simulink model "W1Q1"  (R2020a)
settings: Solver=VariableStepAuto  StartTime=0.0  StopTime=10  FixedStep=10  RelTol=1e-3
values from neighbouring files (symbols this model uses):
  b = 50    [para.m]
  k1 = 50    [para.m]
  k12 = 500    [para.m]
  M1 = 100    [para.m]
  m2 = 5    [para.m]
settings Model: Creator=Vinayak  LastModifiedBy=Vinayak

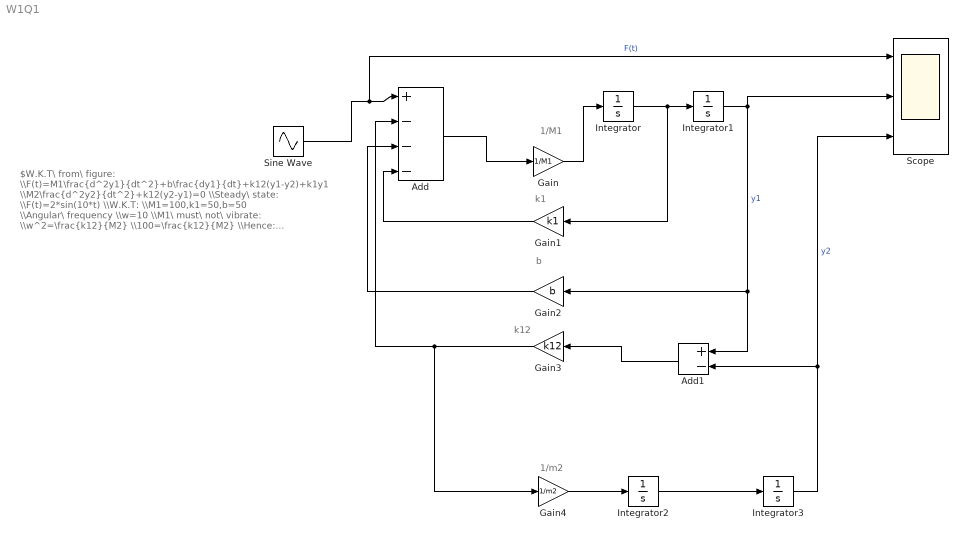
== system W1Q1 ==
  note: $W.K.T\ from\ figure: \\F(t)=M1\frac{d^2y1}{dt^2}+b\frac{dy1}{dt}+k12(y1-y2)+k1y1 \\M2\frac{d^2y2}{dt^2}+k12(y2-y1)=0 \\Steady\ state: \\F(t)=2*sin(10*t) \\W.K.T: \\M1=100,k1=50,b=50 \\Angular\ frequency \\w=10 \\M1\ must\ not\ vibrate: \\w^2=\frac{k12}{M2} \\100=\frac{k12}{M2} \\Hence: \\k12=500,M2=5.$
  note: 1/M1
  note: k1
  note: b
  note: k12
  note: 1/m2
  Add : Sum  Inputs=+---
  Add1 : Sum  Inputs=+-
  Gain : Gain  Gain=1/M1
  Gain1 : Gain  Gain=k1
  Gain2 : Gain  Gain=b
  Gain3 : Gain  Gain=k12
  Gain4 : Gain  Gain=1/m2
  Integrator{,1..3} (4 alike) : Integrator
  Scope : Scope  NumInputPorts=3
  Sine Wave : Sin  Amplitude=2  Frequency=10  SampleTime=0
  wires:
  Sine Wave/1 -> Scope/1, Add/1  "F(t)"
  Add/1 -> Gain/1
  Gain/1 -> Integrator/1
  Integrator/1 -> Gain1/1, Integrator1/1
  Gain1/1 -> Add/4
  Integrator1/1 -> Add1/1, Gain2/1, Scope/2  "y1"
  Gain2/1 -> Add/3
  Add1/1 -> Gain3/1
  Gain3/1 -> Gain4/1, Add/2
  Gain4/1 -> Integrator2/1
  Integrator2/1 -> Integrator3/1
  Integrator3/1 -> Scope/3, Add1/2  "y2"
